simulink model "DENM_Example"  (R2021a)
settings: Solver=VariableStepAuto  StartTime=0.0  StopTime=10.0  RelTol=1e-3
libraries: c2xlib x67
settings Model: EnablePacing=on  Creator=User  LastModifiedBy=User

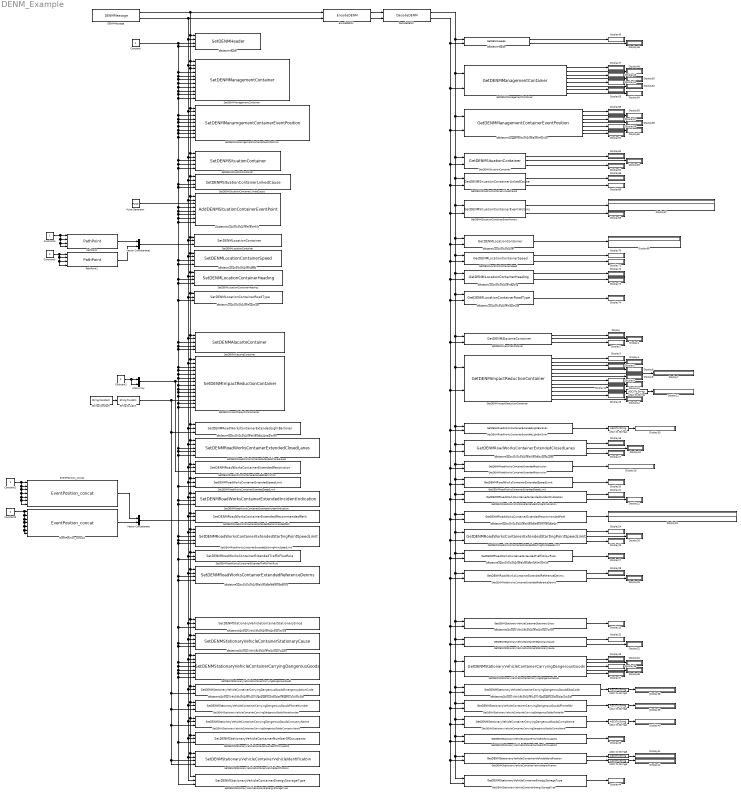
== system DENM_Example ==
  ASCII to String{,1..6} (7 alike) : ASCIIToString
  AddDENMSituationContainerEventPoint : c2xlib/AddDENMSituationContainerEventPoint  SimulateUsing=Code generation
      settings: SourceProductName=C2XLib
  Constant{,1..2,4} (4 alike) : Constant
  Constant3 : Constant  Value=2
  Constant5 : Constant  Value=2
  DENMMessage : c2xlib/DENMMessage  StationID=1  SequenceNumber=1  SimulateUsing=Code generation
      settings: SourceProductName=C2XLib
  DecodeDENM : c2xlib/DecodeDENM  SimulateUsing=Code generation
      settings: SourceProductName=C2XLib
  Display{,1..74} (75 alike) : Display
  EncodeDENM : c2xlib/EncodeDENM  BufferSize=int32( 16384 )  SimulateUsing=Code generation
      settings: SourceProductName=C2XLib
  EventPosition_concat : c2xlib/EventPosition_concat  SimulateUsing=Code generation
      settings: SourceProductName=C2XLib
  EventPosition_concat1 : c2xlib/EventPosition_concat  SimulateUsing=Code generation
      settings: SourceProductName=C2XLib
  GetDENMAlacarteContainer : c2xlib/GetDENMAlacarteContainer  SimulateUsing=Code generation
      settings: SourceProductName=C2XLib
  GetDENMHeader : c2xlib/GetDENMHeader  SimulateUsing=Code generation
      settings: SourceProductName=C2XLib
  GetDENMImpactReductionContainer : c2xlib/GetDENMImpactReductionContainer  PositionOfPillarsSize=2  PositionOfOccupantsSize=32  SimulateUsing=Code generation
      settings: SourceProductName=C2XLib
  GetDENMLocationContainer : c2xlib/GetDENMLocationContainer  NumberTraces=1  TraceLength=2  SimulateUsing=Code generation
      settings: SourceProductName=C2XLib
  GetDENMLocationContainerHeading : c2xlib/GetDENMLocationContainerHeading  SimulateUsing=Code generation
      settings: SourceProductName=C2XLib
  GetDENMLocationContainerRoadType : c2xlib/GetDENMLocationContainerRoadType  SimulateUsing=Code generation
      settings: SourceProductName=C2XLib
  GetDENMLocationContainerSpeed : c2xlib/GetDENMLocationContainerSpeed  SimulateUsing=Code generation
      settings: SourceProductName=C2XLib
  GetDENMManagementContainer : c2xlib/GetDENMManagementContainer  SimulateUsing=Code generation
      settings: SourceProductName=C2XLib
  GetDENMManagementContainerEventPosition : c2xlib/GetDENMManagementContainerEventPosition  SimulateUsing=Code generation
      settings: SourceProductName=C2XLib
  GetDENMRoadWorksContainerExtendedClosedLanes : c2xlib/GetDENMRoadWorksContainerExtendedClosedLanes  SimulateUsing=Code generation
      settings: SourceProductName=C2XLib
  GetDENMRoadWorksContainerExtendedIncidentIndication : c2xlib/GetDENMRoadWorksContainerExtendedIncidentIndication  SimulateUsing=Code generation
      settings: SourceProductName=C2XLib
  GetDENMRoadWorksContainerExtendedLightBarSiren : c2xlib/GetDENMRoadWorksContainerExtendedLightBarSiren  LightBarSirenInUseSize=32  SimulateUsing=Code generation
      settings: SourceProductName=C2XLib
  GetDENMRoadWorksContainerExtendedRecommendedPath : c2xlib/GetDENMRoadWorksContainerExtendedRecommendedPath  ReferencePositionsSize=2  SimulateUsing=Code generation
      settings: SourceProductName=C2XLib
  GetDENMRoadWorksContainerExtendedReferenceDenms : c2xlib/GetDENMRoadWorksContainerExtendedReferenceDenms  ActionIDsSize=1  SimulateUsing=Code generation
      settings: SourceProductName=C2XLib
  GetDENMRoadWorksContainerExtendedRestriction : c2xlib/GetDENMRoadWorksContainerExtendedRestriction  StationTypesSize=2  SimulateUsing=Code generation
      settings: SourceProductName=C2XLib
  GetDENMRoadWorksContainerExtendedSpeedLimit : c2xlib/GetDENMRoadWorksContainerExtendedSpeedLimit  SimulateUsing=Code generation
      settings: SourceProductName=C2XLib
  GetDENMRoadWorksContainerExtendedStartingPointSpeedLimit : c2xlib/GetDENMRoadWorksContainerExtendedStartingPointSpeedLimit  SimulateUsing=Code generation
      settings: SourceProductName=C2XLib
  GetDENMRoadWorksContainerExtendedTrafficFlowRule : c2xlib/GetDENMRoadWorksContainerExtendedTrafficFlowRule  SimulateUsing=Code generation
      settings: SourceProductName=C2XLib
  GetDENMSituationContainer : c2xlib/GetDENMSituationContainer  SimulateUsing=Code generation
      settings: SourceProductName=C2XLib
  GetDENMSituationContainerEventHistory : c2xlib/GetDENMSituationContainerEventHistory  EventHistorySize=2  SimulateUsing=Code generation
      settings: SourceProductName=C2XLib
  GetDENMSituationContainerLinkedCause : c2xlib/GetDENMSituationContainerLinkedCause  SimulateUsing=Code generation
      settings: SourceProductName=C2XLib
  GetDENMStationaryVehicleContainerCarryingDangerousGoods : c2xlib/GetDENMStationaryVehicleContainerCarryingDangerousGoods  SimulateUsing=Code generation
      settings: SourceProductName=C2XLib
  GetDENMStationaryVehicleContainerCarryingDangerousGoodsCompName : c2xlib/GetDENMStationaryVehicleContainerCarryingDangerousGoodsCompName  CompanyNameSize=int32( 16 )  SimulateUsing=Code generation
      settings: SourceProductName=C2XLib
  GetDENMStationaryVehicleContainerCarryingDangerousGoodsEActCode : c2xlib/GetDENMStationaryVehicleContainerCarryingDangerousGoodsEActCode  EmergencyActionCodeSize=int32( 16 )  SimulateUsing=Code generation
      settings: SourceProductName=C2XLib
  GetDENMStationaryVehicleContainerCarryingDangerousGoodsPhoneNbr : c2xlib/GetDENMStationaryVehicleContainerCarryingDangerousGoodsPhoneNbr  PhoneNumberSize=int32( 16 )  SimulateUsing=Code generation
      settings: SourceProductName=C2XLib
  GetDENMStationaryVehicleContainerEnergyStorageType : c2xlib/GetDENMStationaryVehicleContainerEnergyStorageType  SimulateUsing=Code generation
      settings: SourceProductName=C2XLib
  GetDENMStationaryVehicleContainerNumberOfOccupants : c2xlib/GetDENMStationaryVehicleContainerNumberOfOccupants  SimulateUsing=Code generation
      settings: SourceProductName=C2XLib
  GetDENMStationaryVehicleContainerStationaryCause : c2xlib/GetDENMStationaryVehicleContainerStationaryCause  SimulateUsing=Code generation
      settings: SourceProductName=C2XLib
  GetDENMStationaryVehicleContainerStationarySince : c2xlib/GetDENMStationaryVehicleContainerStationarySince  SimulateUsing=Code generation
      settings: SourceProductName=C2XLib
  GetDENMStationaryVehicleContainerVehicleIdentification : c2xlib/GetDENMStationaryVehicleContainerVehicleIdentification  WMInumberSize=int32( 16 )  VDSSize=int32( 16 )  SimulateUsing=Code generation
      settings: SourceProductName=C2XLib
  PathPoint : c2xlib/PathPoint  SimulateUsing=Code generation
      settings: SourceProductName=C2XLib
  PathPoint1 : c2xlib/PathPoint  SimulateUsing=Code generation
      settings: SourceProductName=C2XLib
  Pulse Generator : DiscretePulseGenerator  PulseType=Time based  Period=5  PulseWidth=50  PhaseDelay=1
  SetDENMAlacarteContainer : c2xlib/SetDENMAlacarteContainer  SimulateUsing=Code generation
      settings: SourceProductName=C2XLib
  SetDENMHeader : c2xlib/SetDENMHeader  SimulateUsing=Code generation
      settings: SourceProductName=C2XLib
  SetDENMImpactReductionContainer : c2xlib/SetDENMImpactReductionContainer  SimulateUsing=Code generation
      settings: SourceProductName=C2XLib
  SetDENMLocationContainer : c2xlib/SetDENMLocationContainer  NumberTraces=1  SimulateUsing=Code generation
      settings: SourceProductName=C2XLib
  SetDENMLocationContainerHeading : c2xlib/SetDENMLocationContainerHeading  SimulateUsing=Code generation
      settings: SourceProductName=C2XLib
  SetDENMLocationContainerRoadType : c2xlib/SetDENMLocationContainerRoadType  SimulateUsing=Code generation
      settings: SourceProductName=C2XLib
  SetDENMLocationContainerSpeed : c2xlib/SetDENMLocationContainerSpeed  SimulateUsing=Code generation
      settings: SourceProductName=C2XLib
  SetDENMManagementContainer : c2xlib/SetDENMManagementContainer  SimulateUsing=Code generation
      settings: SourceProductName=C2XLib
  SetDENMManamgementContainerEventPosition : c2xlib/SetDENMManamgementContainerEventPosition  SimulateUsing=Code generation
      settings: SourceProductName=C2XLib
  SetDENMRoadWorksContainerExtendedClosedLanes : c2xlib/SetDENMRoadWorksContainerExtendedClosedLanes  SimulateUsing=Code generation
      settings: SourceProductName=C2XLib
  SetDENMRoadWorksContainerExtendedIncidentIndication : c2xlib/SetDENMRoadWorksContainerExtendedIncidentIndication  SimulateUsing=Code generation
      settings: SourceProductName=C2XLib
  SetDENMRoadWorksContainerExtendedLightBarSiren : c2xlib/SetDENMRoadWorksContainerExtendedLightBarSiren  SimulateUsing=Code generation
      settings: SourceProductName=C2XLib
  SetDENMRoadWorksContainerExtendedRecommendedPath : c2xlib/SetDENMRoadWorksContainerExtendedRecommendedPath  SimulateUsing=Code generation
      settings: SourceProductName=C2XLib
  SetDENMRoadWorksContainerExtendedReferenceDenms : c2xlib/SetDENMRoadWorksContainerExtendedReferenceDenms  NumberActionIDs=1  SimulateUsing=Code generation
      settings: SourceProductName=C2XLib
  SetDENMRoadWorksContainerExtendedRestriction : c2xlib/SetDENMRoadWorksContainerExtendedRestriction  SimulateUsing=Code generation
      settings: SourceProductName=C2XLib
  SetDENMRoadWorksContainerExtendedSpeedLimit : c2xlib/SetDENMRoadWorksContainerExtendedSpeedLimit  SimulateUsing=Code generation
      settings: SourceProductName=C2XLib
  SetDENMRoadWorksContainerExtendedStartingPointSpeedLimit : c2xlib/SetDENMRoadWorksContainerExtendedStartingPointSpeedLimit  SimulateUsing=Code generation
      settings: SourceProductName=C2XLib
  SetDENMRoadWorksContainerExtendedTrafficFlowRule : c2xlib/SetDENMRoadWorksContainerExtendedTrafficFlowRule  SimulateUsing=Code generation
      settings: SourceProductName=C2XLib
  SetDENMSituationContainer : c2xlib/SetDENMSituationContainer  SimulateUsing=Code generation
      settings: SourceProductName=C2XLib
  SetDENMSituationContainerLinkedCause : c2xlib/SetDENMSituationContainerLinkedCause  SimulateUsing=Code generation
      settings: SourceProductName=C2XLib
  SetDENMStationaryVehicleContainerCarryingDangerousGoods : c2xlib/SetDENMStationaryVehicleContainerCarryingDangerousGoods  SimulateUsing=Code generation
      settings: SourceProductName=C2XLib
  SetDENMStationaryVehicleContainerCarryingDangerousGoodsCompanyName : c2xlib/SetDENMStationaryVehicleContainerCarryingDangerousGoodsCompanyName  SimulateUsing=Code generation
      settings: SourceProductName=C2XLib
  SetDENMStationaryVehicleContainerCarryingDangerousGoodsEmergencyActionCode : c2xlib/SetDENMStationaryVehicleContainerCarryingDangerousGoodsEmergencyActionCode  SimulateUsing=Code generation
      settings: SourceProductName=C2XLib
  SetDENMStationaryVehicleContainerCarryingDangerousGoodsPhoneNumber : c2xlib/SetDENMStationaryVehicleContainerCarryingDangerousGoodsPhoneNumber  SimulateUsing=Code generation
      settings: SourceProductName=C2XLib
  SetDENMStationaryVehicleContainerEnergyStorageType : c2xlib/SetDENMStationaryVehicleContainerEnergyStorageType  SimulateUsing=Code generation
      settings: SourceProductName=C2XLib
  SetDENMStationaryVehicleContainerNumberOfOccupants : c2xlib/SetDENMStationaryVehicleContainerNumberOfOccupants  SimulateUsing=Code generation
      settings: SourceProductName=C2XLib
  SetDENMStationaryVehicleContainerStationaryCause : c2xlib/SetDENMStationaryVehicleContainerStationaryCause  SimulateUsing=Code generation
      settings: SourceProductName=C2XLib
  SetDENMStationaryVehicleContainerStationarySince : c2xlib/SetDENMStationaryVehicleContainerStationarySince  SimulateUsing=Code generation
      settings: SourceProductName=C2XLib
  SetDENMStationaryVehicleContainerVehicleIdentificatoin : c2xlib/SetDENMStationaryVehicleContainerVehicleIdentificatoin  SimulateUsing=Code generation
      settings: SourceProductName=C2XLib
  String Constant : StringConstant  String="\"Byte Array\""
  String to ASCII : StringToASCII
  Vector Concatenate : Concatenate
  Vector Concatenate1 : Concatenate
  int32 Array : Concatenate
  wires:
  String Constant/1 -> String to ASCII/1
  Constant1/1 -> int32 Array/2, int32 Array/1
  int32 Array/1 -> SetDENMRoadWorksContainerExtendedRestriction/3, SetDENMImpactReductionContainer/7
  EventPosition_concat/1 -> Vector Concatenate/1
  EventPosition_concat1/1 -> Vector Concatenate/2
  Constant2/1 -> EventPosition_concat/1, EventPosition_concat/4, EventPosition_concat/5, EventPosition_concat/7, EventPosition_concat/6, EventPosition_concat/3, EventPosition_concat/2
  GetDENMAlacarteContainer/2 -> Display1/1
  GetDENMAlacarteContainer/1 -> Display/1
  GetDENMAlacarteContainer/3 -> Display2/1
  GetDENMImpactReductionContainer/3 -> Display5/1
  GetDENMImpactReductionContainer/1 -> Display3/1
  GetDENMImpactReductionContainer/2 -> Display4/1
  GetDENMImpactReductionContainer/4 -> Display6/1
  GetDENMImpactReductionContainer/6 -> Display8/1
  GetDENMImpactReductionContainer/7 -> Display9/1
  GetDENMImpactReductionContainer/5 -> Display7/1
  GetDENMImpactReductionContainer/8 -> Display10/1
  GetDENMImpactReductionContainer/10 -> ASCII to String/1
  GetDENMImpactReductionContainer/11 -> Display13/1
  GetDENMImpactReductionContainer/9 -> Display11/1
  GetDENMImpactReductionContainer/12 -> Display14/1
  ASCII to String/1 -> Display12/1
  GetDENMRoadWorksContainerExtendedLightBarSiren/1 -> ASCII to String1/1
  GetDENMRoadWorksContainerExtendedClosedLanes/1 -> Display16/1
  GetDENMRoadWorksContainerExtendedClosedLanes/3 -> Display17/1
  GetDENMRoadWorksContainerExtendedClosedLanes/2 -> Display18/1
  GetDENMRoadWorksContainerExtendedRestriction/1 -> Display19/1
  GetDENMRoadWorksContainerExtendedSpeedLimit/1 -> Display20/1
  GetDENMRoadWorksContainerExtendedIncidentIndication/1 -> Display21/1
  GetDENMRoadWorksContainerExtendedIncidentIndication/2 -> Display22/1
  GetDENMRoadWorksContainerExtendedRecommendedPath/1 -> Display23/1
  GetDENMRoadWorksContainerExtendedStartingPointSpeedLimit/1 -> Display24/1
  GetDENMRoadWorksContainerExtendedStartingPointSpeedLimit/2 -> Display26/1
  GetDENMRoadWorksContainerExtendedStartingPointSpeedLimit/3 -> Display25/1
  GetDENMRoadWorksContainerExtendedTrafficFlowRule/1 -> Display27/1
  GetDENMRoadWorksContainerExtendedReferenceDenms/2 -> Display29/1
  GetDENMRoadWorksContainerExtendedReferenceDenms/1 -> Display28/1
  ASCII to String1/1 -> Display30/1
  Vector Concatenate/1 -> SetDENMRoadWorksContainerExtendedRecommendedPath/3
  Constant3/1 -> EventPosition_concat1/3, EventPosition_concat1/7, EventPosition_concat1/6, EventPosition_concat1/5, EventPosition_concat1/4, EventPosition_concat1/2, EventPosition_concat1/1
  DENMMessage/2 -> SetDENMHeader/2, SetDENMManagementContainer/2, SetDENMManamgementContainerEventPosition/2, SetDENMSituationContainer/2, SetDENMSituationContainerLinkedCause/2, AddDENMSituationContainerEventPoint/2, SetDENMLocationContainer/2, SetDENMLocationContainerSpeed/2, SetDENMLocationContainerHeading/2, SetDENMLocationContainerRoadType/2, SetDENMRoadWorksContainerExtendedReferenceDenms/2, SetDENMStationaryVehicleContainerNumberOfOccupants/2, SetDENMStationaryVehicleContainerEnergyStorageType/2, SetDENMStationaryVehicleContainerVehicleIdentificatoin/2, SetDENMStationaryVehicleContainerCarryingDangerousGoodsCompanyName/2, SetDENMStationaryVehicleContainerCarryingDangerousGoodsPhoneNumber/2, SetDENMStationaryVehicleContainerCarryingDangerousGoodsEmergencyActionCode/2, SetDENMStationaryVehicleContainerCarryingDangerousGoods/2, SetDENMStationaryVehicleContainerStationaryCause/2, SetDENMStationaryVehicleContainerStationarySince/2, SetDENMRoadWorksContainerExtendedTrafficFlowRule/2, SetDENMRoadWorksContainerExtendedStartingPointSpeedLimit/2, SetDENMRoadWorksContainerExtendedRecommendedPath/2, SetDENMRoadWorksContainerExtendedIncidentIndication/2, SetDENMRoadWorksContainerExtendedSpeedLimit/2, SetDENMRoadWorksContainerExtendedRestriction/2, SetDENMRoadWorksContainerExtendedClosedLanes/2, SetDENMRoadWorksContainerExtendedLightBarSiren/2, SetDENMImpactReductionContainer/2, SetDENMAlacarteContainer/2, EncodeDENM/2
  DENMMessage/1 -> SetDENMHeader/1, SetDENMManagementContainer/1, SetDENMManagementContainer/3, SetDENMManamgementContainerEventPosition/1, SetDENMSituationContainer/1, SetDENMSituationContainerLinkedCause/1, AddDENMSituationContainerEventPoint/1, SetDENMLocationContainer/1, SetDENMLocationContainerSpeed/1, SetDENMLocationContainerHeading/1, SetDENMLocationContainerRoadType/1, SetDENMRoadWorksContainerExtendedReferenceDenms/1, SetDENMStationaryVehicleContainerEnergyStorageType/1, SetDENMStationaryVehicleContainerVehicleIdentificatoin/1, SetDENMStationaryVehicleContainerNumberOfOccupants/1, SetDENMStationaryVehicleContainerCarryingDangerousGoodsCompanyName/1, SetDENMStationaryVehicleContainerCarryingDangerousGoodsPhoneNumber/1, SetDENMStationaryVehicleContainerCarryingDangerousGoodsEmergencyActionCode/1, SetDENMStationaryVehicleContainerCarryingDangerousGoods/1, SetDENMStationaryVehicleContainerStationaryCause/1, SetDENMStationaryVehicleContainerStationarySince/1, SetDENMRoadWorksContainerExtendedTrafficFlowRule/1, SetDENMRoadWorksContainerExtendedStartingPointSpeedLimit/1, SetDENMRoadWorksContainerExtendedRecommendedPath/1, SetDENMRoadWorksContainerExtendedIncidentIndication/1, SetDENMRoadWorksContainerExtendedSpeedLimit/1, SetDENMRoadWorksContainerExtendedRestriction/1, SetDENMRoadWorksContainerExtendedClosedLanes/1, SetDENMRoadWorksContainerExtendedLightBarSiren/1, SetDENMImpactReductionContainer/1, SetDENMAlacarteContainer/1, EncodeDENM/1
  GetDENMStationaryVehicleContainerStationarySince/1 -> Display15/1
  GetDENMStationaryVehicleContainerStationaryCause/1 -> Display31/1
  GetDENMStationaryVehicleContainerStationaryCause/2 -> Display32/1
  GetDENMStationaryVehicleContainerCarryingDangerousGoods/1 -> Display33/1
  GetDENMStationaryVehicleContainerCarryingDangerousGoods/2 -> Display34/1
  GetDENMStationaryVehicleContainerCarryingDangerousGoods/3 -> Display35/1
  GetDENMStationaryVehicleContainerCarryingDangerousGoods/4 -> Display36/1
  GetDENMStationaryVehicleContainerCarryingDangerousGoods/5 -> Display37/1
  ASCII to String2/1 -> Display38/1
  GetDENMStationaryVehicleContainerCarryingDangerousGoodsEActCode/1 -> ASCII to String2/1
  ASCII to String3/1 -> Display39/1
  GetDENMStationaryVehicleContainerCarryingDangerousGoodsPhoneNbr/1 -> ASCII to String3/1
  ASCII to String4/1 -> Display40/1
  GetDENMStationaryVehicleContainerCarryingDangerousGoodsCompName/1 -> ASCII to String4/1
  ASCII to String5/1 -> Display41/1
  GetDENMStationaryVehicleContainerVehicleIdentification/1 -> ASCII to String5/1
  ASCII to String6/1 -> Display42/1
  GetDENMStationaryVehicleContainerVehicleIdentification/2 -> ASCII to String6/1
  GetDENMStationaryVehicleContainerNumberOfOccupants/1 -> Display43/1
  GetDENMStationaryVehicleContainerEnergyStorageType/1 -> Display44/1
  String to ASCII/1 -> SetDENMImpactReductionContainer/12, SetDENMStationaryVehicleContainerCarryingDangerousGoodsEmergencyActionCode/3, SetDENMStationaryVehicleContainerCarryingDangerousGoodsPhoneNumber/3, SetDENMStationaryVehicleContainerCarryingDangerousGoodsCompanyName/3, SetDENMStationaryVehicleContainerVehicleIdentificatoin/3, SetDENMStationaryVehicleContainerVehicleIdentificatoin/4, SetDENMRoadWorksContainerExtendedLightBarSiren/3
  EncodeDENM/1 -> DecodeDENM/1
  EncodeDENM/2 -> DecodeDENM/2
  DecodeDENM/1 -> GetDENMHeader/1, GetDENMManagementContainer/1, GetDENMManagementContainerEventPosition/1, GetDENMSituationContainer/1, GetDENMSituationContainerLinkedCause/1, GetDENMSituationContainerEventHistory/1, GetDENMLocationContainer/1, GetDENMLocationContainerSpeed/1, GetDENMLocationContainerHeading/1, GetDENMLocationContainerRoadType/1, GetDENMStationaryVehicleContainerVehicleIdentification/1, GetDENMStationaryVehicleContainerEnergyStorageType/1, GetDENMStationaryVehicleContainerNumberOfOccupants/1, GetDENMStationaryVehicleContainerCarryingDangerousGoodsCompName/1, GetDENMStationaryVehicleContainerCarryingDangerousGoodsPhoneNbr/1, GetDENMStationaryVehicleContainerCarryingDangerousGoodsEActCode/1, GetDENMStationaryVehicleContainerCarryingDangerousGoods/1, GetDENMStationaryVehicleContainerStationaryCause/1, GetDENMStationaryVehicleContainerStationarySince/1, GetDENMRoadWorksContainerExtendedReferenceDenms/1, GetDENMRoadWorksContainerExtendedTrafficFlowRule/1, GetDENMRoadWorksContainerExtendedStartingPointSpeedLimit/1, GetDENMRoadWorksContainerExtendedRecommendedPath/1, GetDENMRoadWorksContainerExtendedIncidentIndication/1, GetDENMRoadWorksContainerExtendedSpeedLimit/1, GetDENMRoadWorksContainerExtendedRestriction/1, GetDENMRoadWorksContainerExtendedClosedLanes/1, GetDENMRoadWorksContainerExtendedLightBarSiren/1, GetDENMImpactReductionContainer/1, GetDENMAlacarteContainer/1
  DecodeDENM/2 -> GetDENMHeader/2, GetDENMManagementContainer/2, GetDENMManagementContainerEventPosition/2, GetDENMSituationContainer/2, GetDENMSituationContainerLinkedCause/2, GetDENMSituationContainerEventHistory/2, GetDENMLocationContainer/2, GetDENMLocationContainerHeading/2, GetDENMLocationContainerRoadType/2, GetDENMAlacarteContainer/2, GetDENMRoadWorksContainerExtendedLightBarSiren/2, GetDENMRoadWorksContainerExtendedSpeedLimit/2, GetDENMRoadWorksContainerExtendedRecommendedPath/2, GetDENMStationaryVehicleContainerStationaryCause/2, GetDENMStationaryVehicleContainerCarryingDangerousGoods/2, GetDENMStationaryVehicleContainerCarryingDangerousGoodsEActCode/2, GetDENMStationaryVehicleContainerCarryingDangerousGoodsPhoneNbr/2, GetDENMStationaryVehicleContainerCarryingDangerousGoodsCompName/2, GetDENMStationaryVehicleContainerEnergyStorageType/2, GetDENMStationaryVehicleContainerVehicleIdentification/2, GetDENMStationaryVehicleContainerNumberOfOccupants/2, GetDENMStationaryVehicleContainerStationarySince/2, GetDENMRoadWorksContainerExtendedReferenceDenms/2, GetDENMRoadWorksContainerExtendedTrafficFlowRule/2, GetDENMRoadWorksContainerExtendedStartingPointSpeedLimit/2, GetDENMRoadWorksContainerExtendedIncidentIndication/2, GetDENMRoadWorksContainerExtendedRestriction/2, GetDENMRoadWorksContainerExtendedClosedLanes/2, GetDENMImpactReductionContainer/2, GetDENMLocationContainerSpeed/2
  Constant/1 -> SetDENMHeader/3, SetDENMHeader/4, SetDENMManagementContainer/4, SetDENMManagementContainer/5, SetDENMManagementContainer/6, SetDENMManagementContainer/7, SetDENMManagementContainer/8, SetDENMManagementContainer/9, SetDENMManagementContainer/10, SetDENMManagementContainer/11, SetDENMManamgementContainerEventPosition/3, SetDENMManamgementContainerEventPosition/4, SetDENMManamgementContainerEventPosition/5, SetDENMManamgementContainerEventPosition/6, SetDENMManamgementContainerEventPosition/7, SetDENMManamgementContainerEventPosition/8, SetDENMManamgementContainerEventPosition/9, SetDENMSituationContainer/3, SetDENMSituationContainer/4, SetDENMSituationContainer/5, SetDENMSituationContainerLinkedCause/3, SetDENMSituationContainerLinkedCause/4, AddDENMSituationContainerEventPoint/4, AddDENMSituationContainerEventPoint/5, AddDENMSituationContainerEventPoint/6, AddDENMSituationContainerEventPoint/7, AddDENMSituationContainerEventPoint/8, SetDENMLocationContainerSpeed/3, SetDENMLocationContainerSpeed/4, SetDENMLocationContainerHeading/3, SetDENMLocationContainerHeading/4, SetDENMLocationContainerRoadType/3, SetDENMImpactReductionContainer/3, SetDENMImpactReductionContainer/4, SetDENMImpactReductionContainer/5, SetDENMImpactReductionContainer/6, SetDENMImpactReductionContainer/8, SetDENMImpactReductionContainer/9, SetDENMImpactReductionContainer/10, SetDENMImpactReductionContainer/11, SetDENMRoadWorksContainerExtendedReferenceDenms/3, SetDENMRoadWorksContainerExtendedReferenceDenms/4, SetDENMStationaryVehicleContainerStationaryCause/3, SetDENMStationaryVehicleContainerEnergyStorageType/3, SetDENMStationaryVehicleContainerNumberOfOccupants/3, SetDENMStationaryVehicleContainerCarryingDangerousGoods/7, SetDENMStationaryVehicleContainerCarryingDangerousGoods/6, SetDENMStationaryVehicleContainerCarryingDangerousGoods/5, SetDENMStationaryVehicleContainerCarryingDangerousGoods/4, SetDENMStationaryVehicleContainerCarryingDangerousGoods/3, SetDENMStationaryVehicleContainerStationaryCause/4, SetDENMStationaryVehicleContainerStationarySince/3, SetDENMRoadWorksContainerExtendedTrafficFlowRule/3, SetDENMRoadWorksContainerExtendedStartingPointSpeedLimit/5, SetDENMRoadWorksContainerExtendedStartingPointSpeedLimit/4, SetDENMRoadWorksContainerExtendedStartingPointSpeedLimit/3, SetDENMRoadWorksContainerExtendedIncidentIndication/4, SetDENMRoadWorksContainerExtendedIncidentIndication/3, SetDENMRoadWorksContainerExtendedSpeedLimit/3, SetDENMRoadWorksContainerExtendedClosedLanes/5, SetDENMRoadWorksContainerExtendedClosedLanes/4, SetDENMRoadWorksContainerExtendedClosedLanes/3, SetDENMImpactReductionContainer/14, SetDENMImpactReductionContainer/13, SetDENMAlacarteContainer/5, SetDENMAlacarteContainer/4, SetDENMAlacarteContainer/3
  Pulse Generator/1 -> AddDENMSituationContainerEventPoint/3
  GetDENMHeader/1 -> Display45/1
  GetDENMHeader/2 -> Display46/1
  GetDENMManagementContainer/1 -> Display47/1
  GetDENMManagementContainer/3 -> Display49/1
  GetDENMManagementContainer/2 -> Display48/1
  GetDENMManagementContainer/4 -> Display50/1
  GetDENMManagementContainer/5 -> Display51/1
  GetDENMManagementContainer/6 -> Display52/1
  GetDENMManagementContainer/7 -> Display53/1
  GetDENMManagementContainer/8 -> Display54/1
  GetDENMManagementContainerEventPosition/1 -> Display55/1
  GetDENMManagementContainerEventPosition/2 -> Display56/1
  GetDENMManagementContainerEventPosition/3 -> Display57/1
  GetDENMManagementContainerEventPosition/4 -> Display58/1
  GetDENMManagementContainerEventPosition/5 -> Display59/1
  GetDENMManagementContainerEventPosition/6 -> Display60/1
  GetDENMManagementContainerEventPosition/7 -> Display61/1
  GetDENMSituationContainerLinkedCause/2 -> Display66/1
  GetDENMSituationContainerLinkedCause/1 -> Display65/1
  GetDENMSituationContainer/3 -> Display64/1
  GetDENMSituationContainer/2 -> Display63/1
  GetDENMSituationContainer/1 -> Display62/1
  GetDENMSituationContainerEventHistory/2 -> Display68/1
  GetDENMSituationContainerEventHistory/1 -> Display67/1
  GetDENMLocationContainer/1 -> Display69/1
  GetDENMLocationContainerSpeed/2 -> Display71/1
  GetDENMLocationContainerSpeed/1 -> Display70/1
  GetDENMLocationContainerHeading/2 -> Display73/1
  GetDENMLocationContainerHeading/1 -> Display72/1
  GetDENMLocationContainerRoadType/1 -> Display74/1
  Vector Concatenate1/1 -> SetDENMLocationContainer/3
  PathPoint/1 -> Vector Concatenate1/1
  PathPoint1/1 -> Vector Concatenate1/2
  Constant4/1 -> PathPoint/4, PathPoint/3, PathPoint/2, PathPoint/1
  Constant5/1 -> PathPoint1/4, PathPoint1/3, PathPoint1/2, PathPoint1/1
